simulink model "drone_model"  (R2023a)
settings: Solver=VariableStepAuto  StartTime=0.0  StopTime=10.0  RelTol=1e-3
values from neighbouring files (symbols this model uses):
  g = 9.81    [verify_dynamics.m]
  l = 1    [verify_dynamics.m]
  m = 2    [verify_dynamics.m]
libraries: shared6dof x1, sharedtransform x1, SignalEditorBlockLib x1
settings Model: Creator=timme  LastModifiedBy=timme

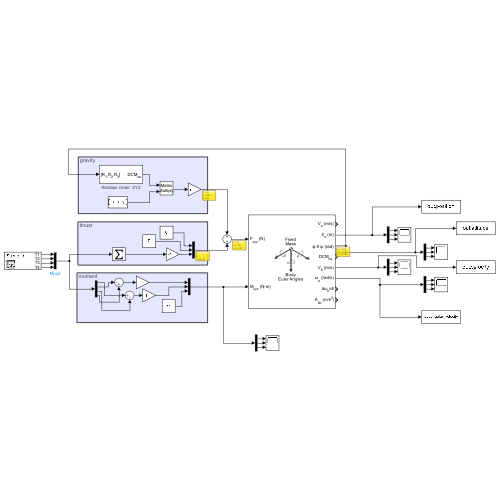
[thumbnail: Simulink's stored preview of the top-level diagram]
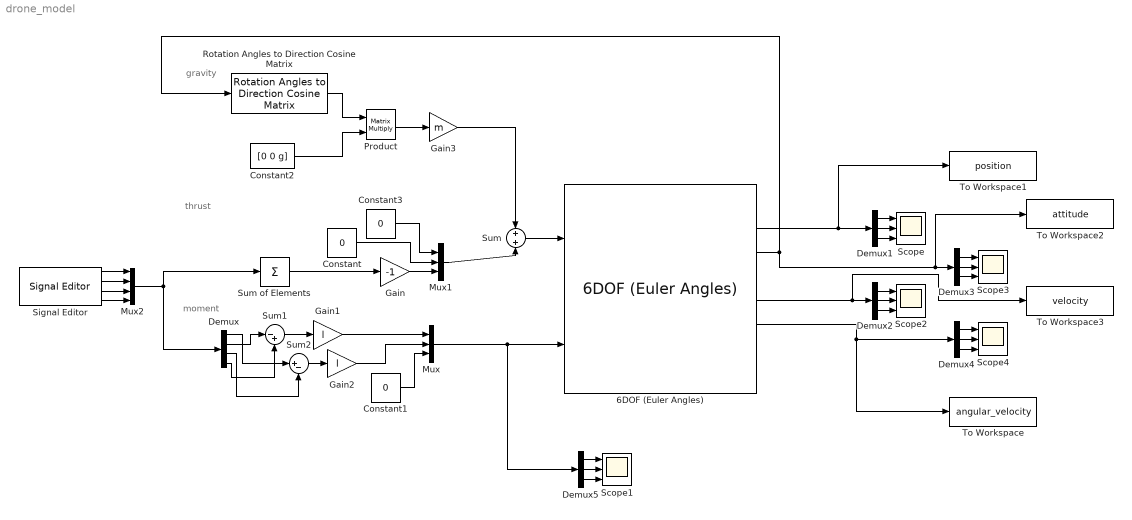
== system drone_model ==
  note: moment
  note: thrust
  note: gravity
  6DOF (Euler Angles) : shared6dof/6DOF (Euler Angles)  units=Metric (MKS)  mtype=Fixed  rep=Euler Angles  xme_0=[0 0 0]  Vm_0=[0 0 0]  eul_0=[0 0 0]  pm_0=[0 0 0]  mass_0=m  mass_e=0.5  mass_f=2.0  inertia=I  inertia_e=eye(3)  inertia_f=2*eye(3)  k_quat=1.0  vre_flag=on  abi_flag=off  aMode=0  xme_statename=''  Vm_statename=''  eul_statename=''  quat_statename=''  pm_statename=''  mass_statename=''
  Constant : Constant  Value=0
  Constant1 : Constant  Value=0
  Constant2 : Constant  Value=[0 0 g]
  Constant3 : Constant  Value=0
  Demux : Demux
  Demux{1..5} (5 alike) : Demux  Outputs=3
  Gain : Gain  Gain=-1
  Gain1 : Gain  Gain=l
  Gain2 : Gain  Gain=l
  Gain3 : Gain  Gain=m
  Mux : Mux  Inputs=3
  Mux1 : Mux  Inputs=3
  Mux2 : Mux
  Product : Product  Multiplication=Matrix(*)
  Rotation Angles to Direction Cosine Matrix : sharedtransform/Rotation Angles to Direction Cosine Matrix  rotationOrder=XYZ  aMode=aMode
  Scope{,1..4} (5 alike) : Scope  NumInputPorts=3
  Signal Editor : SignalEditorBlockLib/Signal Editor  FileName=test_input_2.mat  ActiveScenario=Scenario  ActiveSignal=T1  IsBus=off  OutputBusObjectStr=Bus: BusObject  SampleTime=0  Interpolate=off  ZeroCross=off  OutputAfterFinalValue=Setting to zero  Unit=inherit  PreserveSignalName=on  ApplySigPropsToAllScenarios=on
  Sum : Sum  Inputs=+|+
  Sum of Elements : Sum  Inputs=+
  Sum1 : Sum  Inputs=|-+
  Sum2 : Sum  Inputs=|+-
  To Workspace : ToWorkspace  VariableName=angular_velocity  SaveFormat=Timeseries  SampleTime=0.01
      settings: Decimation=2
  To Workspace1 : ToWorkspace  VariableName=position  SaveFormat=Timeseries  SampleTime=0.01
      settings: Decimation=2
  To Workspace2 : ToWorkspace  VariableName=attitude  SaveFormat=Timeseries  SampleTime=0.01
      settings: Decimation=2
  To Workspace3 : ToWorkspace  VariableName=velocity  SaveFormat=Timeseries  SampleTime=0.01
      settings: Decimation=2
  wires:
  Mux2/1 -> Sum of Elements/1, Demux/1
  Rotation Angles to Direction Cosine Matrix/1 -> Product/1
  Constant2/1 -> Product/2
  Sum/1 -> 6DOF (Euler Angles)/1
  Product/1 -> Gain3/1
  Sum of Elements/1 -> Gain/1
  Gain/1 -> Mux1/3
  Mux/1 -> Demux5/1, 6DOF (Euler Angles)/2
  Constant1/1 -> Mux/3
  Demux/4 -> Sum1/2
  Demux/2 -> Sum1/1
  Sum1/1 -> Gain1/1
  Gain1/1 -> Mux/1
  Demux/1 -> Sum2/1
  Demux/3 -> Sum2/2
  Sum2/1 -> Gain2/1
  Gain2/1 -> Mux/2
  6DOF (Euler Angles)/2 -> To Workspace1/1, Demux1/1
  Mux1/1 -> Sum/2
  Constant/1 -> Mux1/2
  Constant3/1 -> Mux1/1
  Gain3/1 -> Sum/1
  Demux1/2 -> Scope/2
  Demux1/3 -> Scope/3
  Demux1/1 -> Scope/1
  Demux2/2 -> Scope2/2
  6DOF (Euler Angles)/5 -> To Workspace3/1, Demux2/1
  Demux2/3 -> Scope2/3
  Demux2/1 -> Scope2/1
  Signal Editor/1 -> Mux2/1
  Signal Editor/2 -> Mux2/2
  Signal Editor/3 -> Mux2/3
  Signal Editor/4 -> Mux2/4
  Demux3/2 -> Scope3/2
  Demux3/3 -> Scope3/3
  Demux3/1 -> Scope3/1
  6DOF (Euler Angles)/6 -> Demux4/1, To Workspace/1
  Demux4/2 -> Scope4/2
  Demux4/1 -> Scope4/1
  Demux4/3 -> Scope4/3
  6DOF (Euler Angles)/3 -> To Workspace2/1, Demux3/1, Rotation Angles to Direction Cosine Matrix/1
  Demux5/3 -> Scope1/3
  Demux5/1 -> Scope1/1
  Demux5/2 -> Scope1/2
